simulink model "MdXXHolderChk"  (R2024b)
settings: Solver=FixedStepDiscrete  StartTime=0.0  StopTime=10.0  FixedStep=0.01  RelTol=1e-3
undefined symbols (not defined in the file or in its folder): KeSMSwAcsMd32SecRwLtStBkReclnUpwdDnwdPos1_Val, KeSMSwAcsMd53SecRwRtStBkReclnUpwdDnwdPos1_Val, SeatChldLkSt
libraries: simulink x41
(part 1 of 5)
settings Model: Creator=sn2xws  LastModifiedBy=sn55gm
settings Model: ModifiedHistory=|
  | 2024.7.9 V3.0.0 557模式流程V1.9
  | 2024.8.22 V3.0.1 修改Md8 Md9 退出逻辑
  | 2024.8.27 V3.0.2 Md1退出逻辑增加
  | 2024.8.28 V3.0.3 修正设置的bit位
  | 2024.10.25 V3.0.4 6s版 vipR不看三左儿童锁
  | 2024.10.29 V3.0.5 新增三排儿童锁逻辑
  | 2024.11.20 V3.0.6 md8，md9 只有7s版本需要看二排儿童锁
  | 2024.11.26 V3.0.7 Md28 只有7s版本需要看三排左儿童锁，Md27需要看三排童锁
  | 2024.12.11 V3.0.8 CR955881
  | 2024.12.23 V3.8.0 CR963463 二三排复位模式和大四座模式调用前提条件优化
  | 2025.3.5 V3.9.0 Bug 998190 7s 2L儿童锁Lock状态，2L靠背为0%，2R靠背大于31.7%，VCU调用mode 8，StPassCmprtMd_Md8_VCU_RclRspStat= error（应为successfully）
  | 2025.5.13 V3.12.0 Md11，md13，md32,md53童锁条件遗漏
  | 2025.5.14 V3.12.1 bug 1038602童锁时不应该动靠背
  | 2025.5.20 V3.12.2 bug 1038602童锁时不应该动靠背
  | 25.7.2 V3.13.0 新增Md61 Md62
settings SolverCC: AlgebraicLoopSolver=TrustRegion
settings DataIOCC: SaveFormat=StructureWithTime  ReturnWorkspaceOutputs=off
settings OptimizationCC: DefaultParameterBehavior=Inlined  EnhancedBackFolding=on  PassReuseOutputArgsAs=Individual arguments  ZeroExternalMemoryAtStartup=off  ZeroInternalMemoryAtStartup=off  OptimizeBlockOrder=speed  DifferentSizesBufferReuse=on  OptimizationCustomize=off  EfficientTunableParamExpr=on
settings DebuggingCC: ParameterTunabilityLossMsg=error  UnconnectedInputMsg=warning  UnconnectedOutputMsg=warning  UnconnectedLineMsg=warning  ArithmeticOperatorsInVariantConditions=warning
settings ModelReferenceCC: EnableRefExpFcnMdlSchedulingChecks=on
settings SFSimCC: MATLABDynamicMemAlloc=off  CustomCodeUndefinedFunction=UseInterfaceOnly
settings RTWCC: Description=AUTOSAR  SystemTargetFile=autosar.tlc  GenCodeOnly=on  TemplateMakefile=ert_default_tmf  GenerateReport=on  IncludeHyperlinkInReport=on  LaunchReport=on  DataTypeReplacement=CDataTypesFixedWidth  GenerateTraceInfo=on  GenerateTraceReport=on  GenerateTraceReportSl=on  GenerateTraceReportSf=on  GenerateTraceReportEml=on  GPUComputeCapability=3.5
settings CodeAppCC: ForceParamTrailComments=on  IgnoreCustomStorageClasses=off  OperatorAnnotations=on  SimulinkDataObjDesc=on  SFDataObjDesc=on  InsertBlockDesc=on
settings STFCustomTargetCC: TargetLangStandard=C99 (ISO)  MultiwordLength=256  ParMdlRefBuildCompliant=on  CompOptLevelCompliant=on  IncludeMdlTerminateFcn=off  CombineOutputUpdateFcns=on  SuppressErrorStatus=on  ERTCustomFileBanners=on  SupportNonFinite=off  SupportComplex=off  SupportContinuousTime=off  SupportNonInlinedSFcns=off  RemoveResetFunc=on  MATLABClassNameForMDSCustomization=Simulink.SoftwareTarget.ERTCustomization  AutosarCompliant=on  UseToolchainInfoCompliant=on  LookupTableObjectStructAxisOrder=2,1,3,4,...  LUTObjectStructOrderEvenSpacing=Size,Table,Breakpoints  SystemTargetFile=autosar.tlc
settings ERTTargetCC: TargetLangStandard=C99 (ISO)  ConcurrentExecutionCompliant=off  IncludeMdlTerminateFcn=off  SuppressErrorStatus=on  SupportNonFinite=off  SupportComplex=off  ModelStepFunctionPrototypeControlCompliant=off  CPPClassGenCompliant=off  AutosarCompliant=on  LookupTableObjectStructAxisOrder=2,1,3,4,...  LUTObjectStructOrderEvenSpacing=Size,Table,Breakpoints  ERTCustomFileTemplate=example_file_process.tlc  ERTFilePackagingFormat=Compact  BooleanTrueId=TRUE  BooleanFalseId=FALSE  DynamicArrayContainerType=coder::array

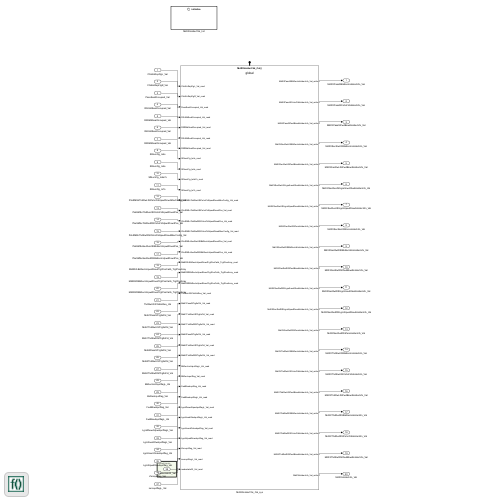
[thumbnail: Simulink's stored preview of the top-level diagram]
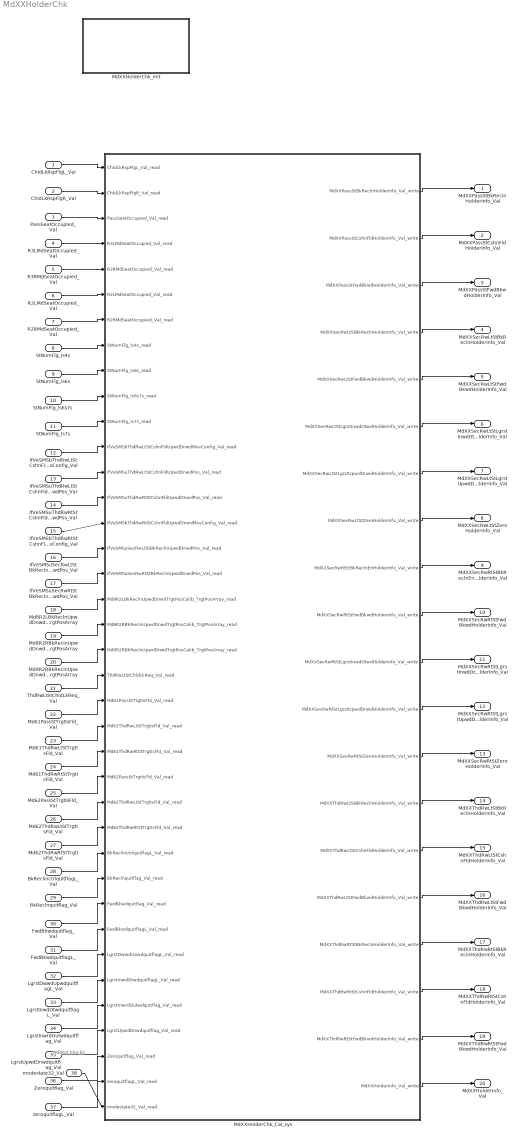
== system MdXXHolderChk ==
  note: Added blocks
  ChldLkRspFlgL_Val : Inport  OutDataTypeStr=boolean  PortDimensions=1
  ChldLkRspFlgR_Val : Inport  Port=2  OutDataTypeStr=boolean  PortDimensions=1
  PassSeatOccupied_Val : Inport  Port=3  OutDataTypeStr=boolean  PortDimensions=1
  R3LMdSeatOccupied_Val : Inport  Port=4  OutDataTypeStr=boolean  PortDimensions=1
  R3RMdSeatOccupied_Val : Inport  Port=5  OutDataTypeStr=boolean  PortDimensions=1
  R2LMdSeatOccupied_Val : Inport  Port=6  OutDataTypeStr=boolean  PortDimensions=1
  R2RMdSeatOccupied_Val : Inport  Port=7  OutDataTypeStr=boolean  PortDimensions=1
  StNumFlg_Is4s : Inport  Port=8  OutDataTypeStr=boolean  PortDimensions=1
  StNumFlg_Is6s : Inport  Port=9  OutDataTypeStr=boolean  PortDimensions=1
  StNumFlg_Is6s7s : Inport  Port=10  OutDataTypeStr=boolean  PortDimensions=1
  StNumFlg_Is7s : Inport  Port=11  OutDataTypeStr=boolean  PortDimensions=1
  IfVeSMSbThdRwLtStCshnFldUpwdDnwdMovConfig_Val : Inport  Port=12  OutDataTypeStr=boolean  PortDimensions=1
  IfVeSMSuThdRwLtStCshnFldUpwdDnwdPos_Val : Inport  Port=13  OutDataTypeStr=uint16  PortDimensions=1
  IfVeSMSuThdRwRtStCshnFldUpwdDnwdPos_Val : Inport  Port=14  OutDataTypeStr=uint16  PortDimensions=1
  IfVeSMSbThdRwRtStCshnFldUpwdDnwdMovConfig_Val : Inport  Port=15  OutDataTypeStr=boolean  PortDimensions=1
  IfVeSMSuSecRwLtStBkReclnUpwdDnwdPos_Val : Inport  Port=16  OutDataTypeStr=uint16  PortDimensions=1
  IfVeSMSuSecRwRtStBkReclnUpwdDnwdPos_Val : Inport  Port=17  OutDataTypeStr=uint16  PortDimensions=1
  Md8R2LBkReclnUpwdDnwdTrgtPosCalib_TrgtPosArray : Inport  Description=|  Port=18  OutDataTypeStr=uint16  PortDimensions=3
      | 0:Pos
      | 1:Max
      | 2:Min
  Md8R2RBkReclnUpwdDnwdTrgtPosCalib_TrgtPosArray : Inport  Description=|  Port=19  OutDataTypeStr=uint16  PortDimensions=3
      | 0:Pos
      | 1:Max
      | 2:Min
  Md9R2RBkReclnUpwdDnwdTrgtPosCalib_TrgtPosArray : Inport  Description=|  Port=20  OutDataTypeStr=uint16  PortDimensions=3
      | 0:Pos
      | 1:Max
      | 2:Min
  ThdRwLtStChldLkReq_Val : Inport  Port=21  OutDataTypeStr=Enum: SeatChldLkSt  PortDimensions=1
  Md61PassStTrgtIsFld_Val : Inport  Port=22  OutDataTypeStr=boolean  PortDimensions=1
  Md61ThdRwLtStTrgtIsFld_Val : Inport  Port=23  OutDataTypeStr=boolean  PortDimensions=1
  Md61ThdRwRtStTrgtIsFld_Val : Inport  Port=24  OutDataTypeStr=boolean  PortDimensions=1
  Md62PassStTrgtIsFld_Val : Inport  Port=25  OutDataTypeStr=boolean  PortDimensions=1
  Md62ThdRwLtStTrgtIsFld_Val : Inport  Port=26  OutDataTypeStr=boolean  PortDimensions=1
  Md62ThdRwRtStTrgtIsFld_Val : Inport  Port=27  OutDataTypeStr=boolean  PortDimensions=1
  BkReclinctrlquitflagL_Val : Inport  Port=28  OutDataTypeStr=boolean  PortDimensions=1
  BkReclnquitflag_Val : Inport  Port=29  OutDataTypeStr=boolean  PortDimensions=1
  FwdBkwdquitflag_Val : Inport  Port=30  OutDataTypeStr=boolean  PortDimensions=1
  FwdBkwdquitflagL_Val : Inport  Port=31  OutDataTypeStr=boolean  PortDimensions=1
  LgrstDwwdUpwdquitflagL_Val : Inport  Port=32  OutDataTypeStr=boolean  PortDimensions=1
  LgrstInwdOtwdquitflagL_Val : Inport  Port=33  OutDataTypeStr=boolean  PortDimensions=1
  LgrstInwrdOutwdquitflag_Val : Inport  Port=34  OutDataTypeStr=boolean  PortDimensions=1
  LgrstUpwdDnwdquitflag_Val : Inport  Port=35  OutDataTypeStr=boolean  PortDimensions=1
  Zeroquitflag_Val : Inport  Port=36  OutDataTypeStr=boolean  PortDimensions=1
  zeroquitflagL_Val : Inport  Port=37  OutDataTypeStr=boolean  PortDimensions=1
  modestate32_Val : Inport  Port=38  OutDataTypeStr=uint32  PortDimensions=1
  MdXXHolderChk_Cal_sys : Subsystem
  MdXXHolderChk_Init : Subsystem
  MdXXPassStBkReclnHolderInfo_Val : Outport  OutDataTypeStr=uint32  PortDimensions=1  VectorParamsAs1DForOutWhenUnconnected=off
  MdXXPassStCshnFldHolderInfo_Val : Outport  Port=2  OutDataTypeStr=uint32  PortDimensions=1  VectorParamsAs1DForOutWhenUnconnected=off
  MdXXPassStFwdBkwdHolderInfo_Val : Outport  Port=3  OutDataTypeStr=uint32  PortDimensions=1  VectorParamsAs1DForOutWhenUnconnected=off
  MdXXSecRwLtStBkReclnHolderInfo_Val : Outport  Port=4  OutDataTypeStr=uint32  PortDimensions=1  VectorParamsAs1DForOutWhenUnconnected=off
  MdXXSecRwLtStFwdBkwdHolderInfo_Val : Outport  Port=5  OutDataTypeStr=uint32  PortDimensions=1  VectorParamsAs1DForOutWhenUnconnected=off
  MdXXSecRwLtStLgrstInwdOtwdHolderInfo_Val : Outport  Port=6  OutDataTypeStr=uint32  PortDimensions=1  VectorParamsAs1DForOutWhenUnconnected=off
  MdXXSecRwLtStLgrstUpwdDnwdHolderInfo_Val : Outport  Port=7  OutDataTypeStr=uint32  PortDimensions=1  VectorParamsAs1DForOutWhenUnconnected=off
  MdXXSecRwLtStZeroHolderInfo_Val : Outport  Port=8  OutDataTypeStr=uint32  PortDimensions=1  VectorParamsAs1DForOutWhenUnconnected=off
  MdXXSecRwRtStBkReclnEnHolderInfo_Val : Outport  Port=9  OutDataTypeStr=uint32  PortDimensions=1  VectorParamsAs1DForOutWhenUnconnected=off
  MdXXSecRwRtStFwdBkwdHolderInfo_Val : Outport  Port=10  OutDataTypeStr=uint32  PortDimensions=1  VectorParamsAs1DForOutWhenUnconnected=off
  MdXXSecRwRtStLgrstInwdOtwdHolderInfo_Val : Outport  Port=11  OutDataTypeStr=uint32  PortDimensions=1  VectorParamsAs1DForOutWhenUnconnected=off
  MdXXSecRwRtStLgrstUpwdDnwdHolderInfo_Val : Outport  Port=12  OutDataTypeStr=uint32  PortDimensions=1  VectorParamsAs1DForOutWhenUnconnected=off
  MdXXSecRwRtStZeroHolderInfo_Val : Outport  Port=13  OutDataTypeStr=uint32  PortDimensions=1  VectorParamsAs1DForOutWhenUnconnected=off
  MdXXThdRwLtStBkReclnHolderInfo_Val : Outport  Port=14  OutDataTypeStr=uint32  PortDimensions=1  VectorParamsAs1DForOutWhenUnconnected=off
  MdXXThdRwLtStCshnFldHolderInfo_Val : Outport  Port=15  OutDataTypeStr=uint32  PortDimensions=1  VectorParamsAs1DForOutWhenUnconnected=off
  MdXXThdRwLtStFwdBkwdHolderInfo_Val : Outport  Port=16  OutDataTypeStr=uint32  PortDimensions=1  VectorParamsAs1DForOutWhenUnconnected=off
  MdXXThdRwRtStBkReclnHolderInfo_Val : Outport  Port=17  OutDataTypeStr=uint32  PortDimensions=1  VectorParamsAs1DForOutWhenUnconnected=off
  MdXXThdRwRtStCshnFldHolderInfo_Val : Outport  Port=18  OutDataTypeStr=uint32  PortDimensions=1  VectorParamsAs1DForOutWhenUnconnected=off
  MdXXThdRwRtStFwdBkwdHolderInfo_Val : Outport  Port=19  OutDataTypeStr=uint32  PortDimensions=1  VectorParamsAs1DForOutWhenUnconnected=off
  MdXXHolderInfo_Val : Outport  Port=20  OutDataTypeStr=uint32  PortDimensions=1  VectorParamsAs1DForOutWhenUnconnected=off
  wires:
  ChldLkRspFlgL_Val/1 -> MdXXHolderChk_Cal_sys/1(ChldLkRspFlgL_Val_read)
  ChldLkRspFlgR_Val/1 -> MdXXHolderChk_Cal_sys/2(ChldLkRspFlgR_Val_read)
  PassSeatOccupied_Val/1 -> MdXXHolderChk_Cal_sys/3(PassSeatOccupied_Val_read)
  R3LMdSeatOccupied_Val/1 -> MdXXHolderChk_Cal_sys/4(R3LMdSeatOccupied_Val_read)
  R3RMdSeatOccupied_Val/1 -> MdXXHolderChk_Cal_sys/5(R3RMdSeatOccupied_Val_read)
  MdXXHolderChk_Cal_sys/1(MdXXPassStBkReclnHolderInfo_Val_write) -> MdXXPassStBkReclnHolderInfo_Val/1
  MdXXHolderChk_Cal_sys/2(MdXXPassStCshnFldHolderInfo_Val_write) -> MdXXPassStCshnFldHolderInfo_Val/1
  MdXXHolderChk_Cal_sys/3(MdXXPassStFwdBkwdHolderInfo_Val_write) -> MdXXPassStFwdBkwdHolderInfo_Val/1
  MdXXHolderChk_Cal_sys/4(MdXXSecRwLtStBkReclnHolderInfo_Val_write) -> MdXXSecRwLtStBkReclnHolderInfo_Val/1
  MdXXHolderChk_Cal_sys/5(MdXXSecRwLtStFwdBkwdHolderInfo_Val_write) -> MdXXSecRwLtStFwdBkwdHolderInfo_Val/1
  MdXXHolderChk_Cal_sys/6(MdXXSecRwLtStLgrstInwdOtwdHolderInfo_Val_write) -> MdXXSecRwLtStLgrstInwdOtwdHolderInfo_Val/1
  MdXXHolderChk_Cal_sys/7(MdXXSecRwLtStLgrstUpwdDnwdHolderInfo_Val_write) -> MdXXSecRwLtStLgrstUpwdDnwdHolderInfo_Val/1
  MdXXHolderChk_Cal_sys/8(MdXXSecRwLtStZeroHolderInfo_Val_write) -> MdXXSecRwLtStZeroHolderInfo_Val/1
  MdXXHolderChk_Cal_sys/9(MdXXSecRwRtStBkReclnEnHolderInfo_Val_write) -> MdXXSecRwRtStBkReclnEnHolderInfo_Val/1
  MdXXHolderChk_Cal_sys/10(MdXXSecRwRtStFwdBkwdHolderInfo_Val_write) -> MdXXSecRwRtStFwdBkwdHolderInfo_Val/1
  MdXXHolderChk_Cal_sys/11(MdXXSecRwRtStLgrstInwdOtwdHolderInfo_Val_write) -> MdXXSecRwRtStLgrstInwdOtwdHolderInfo_Val/1
  MdXXHolderChk_Cal_sys/12(MdXXSecRwRtStLgrstUpwdDnwdHolderInfo_Val_write) -> MdXXSecRwRtStLgrstUpwdDnwdHolderInfo_Val/1
  MdXXHolderChk_Cal_sys/13(MdXXSecRwRtStZeroHolderInfo_Val_write) -> MdXXSecRwRtStZeroHolderInfo_Val/1
  MdXXHolderChk_Cal_sys/14(MdXXThdRwLtStBkReclnHolderInfo_Val_write) -> MdXXThdRwLtStBkReclnHolderInfo_Val/1
  MdXXHolderChk_Cal_sys/15(MdXXThdRwLtStCshnFldHolderInfo_Val_write) -> MdXXThdRwLtStCshnFldHolderInfo_Val/1
  MdXXHolderChk_Cal_sys/16(MdXXThdRwLtStFwdBkwdHolderInfo_Val_write) -> MdXXThdRwLtStFwdBkwdHolderInfo_Val/1
  MdXXHolderChk_Cal_sys/17(MdXXThdRwRtStBkReclnHolderInfo_Val_write) -> MdXXThdRwRtStBkReclnHolderInfo_Val/1
  MdXXHolderChk_Cal_sys/18(MdXXThdRwRtStCshnFldHolderInfo_Val_write) -> MdXXThdRwRtStCshnFldHolderInfo_Val/1
  MdXXHolderChk_Cal_sys/19(MdXXThdRwRtStFwdBkwdHolderInfo_Val_write) -> MdXXThdRwRtStFwdBkwdHolderInfo_Val/1
  R2LMdSeatOccupied_Val/1 -> MdXXHolderChk_Cal_sys/6(R2LMdSeatOccupied_Val_read)
  R2RMdSeatOccupied_Val/1 -> MdXXHolderChk_Cal_sys/7(R2RMdSeatOccupied_Val_read)
  StNumFlg_Is4s/1 -> MdXXHolderChk_Cal_sys/8(StNumFlg_Is4s_read)
  StNumFlg_Is6s/1 -> MdXXHolderChk_Cal_sys/9(StNumFlg_Is6s_read)
  StNumFlg_Is6s7s/1 -> MdXXHolderChk_Cal_sys/10(StNumFlg_Is6s7s_read)
  StNumFlg_Is7s/1 -> MdXXHolderChk_Cal_sys/11(StNumFlg_Is7s_read)
  IfVeSMSbThdRwLtStCshnFldUpwdDnwdMovConfig_Val/1 -> MdXXHolderChk_Cal_sys/12(IfVeSMSbThdRwLtStCshnFldUpwdDnwdMovConfig_Val_read)
  IfVeSMSuThdRwLtStCshnFldUpwdDnwdPos_Val/1 -> MdXXHolderChk_Cal_sys/13(IfVeSMSuThdRwLtStCshnFldUpwdDnwdPos_Val_read)
  IfVeSMSuThdRwRtStCshnFldUpwdDnwdPos_Val/1 -> MdXXHolderChk_Cal_sys/14(IfVeSMSuThdRwRtStCshnFldUpwdDnwdPos_Val_read)
  IfVeSMSbThdRwRtStCshnFldUpwdDnwdMovConfig_Val/1 -> MdXXHolderChk_Cal_sys/15(IfVeSMSbThdRwRtStCshnFldUpwdDnwdMovConfig_Val_read)
  IfVeSMSuSecRwLtStBkReclnUpwdDnwdPos_Val/1 -> MdXXHolderChk_Cal_sys/16(IfVeSMSuSecRwLtStBkReclnUpwdDnwdPos_Val_read)
  IfVeSMSuSecRwRtStBkReclnUpwdDnwdPos_Val/1 -> MdXXHolderChk_Cal_sys/17(IfVeSMSuSecRwRtStBkReclnUpwdDnwdPos_Val_read)
  Md8R2LBkReclnUpwdDnwdTrgtPosCalib_TrgtPosArray/1 -> MdXXHolderChk_Cal_sys/18(Md8R2LBkReclnUpwdDnwdTrgtPosCalib_TrgtPosArray_read)
  Md8R2RBkReclnUpwdDnwdTrgtPosCalib_TrgtPosArray/1 -> MdXXHolderChk_Cal_sys/19(Md8R2RBkReclnUpwdDnwdTrgtPosCalib_TrgtPosArray_read)
  Md9R2RBkReclnUpwdDnwdTrgtPosCalib_TrgtPosArray/1 -> MdXXHolderChk_Cal_sys/20(Md9R2RBkReclnUpwdDnwdTrgtPosCalib_TrgtPosArray_read)
  ThdRwLtStChldLkReq_Val/1 -> MdXXHolderChk_Cal_sys/21(ThdRwLtStChldLkReq_Val_read)
  MdXXHolderChk_Cal_sys/20(MdXXHolderInfo_Val_write) -> MdXXHolderInfo_Val/1
  Md61PassStTrgtIsFld_Val/1 -> MdXXHolderChk_Cal_sys/22(Md61PassStTrgtIsFld_Val_read)
  Md61ThdRwLtStTrgtIsFld_Val/1 -> MdXXHolderChk_Cal_sys/23(Md61ThdRwLtStTrgtIsFld_Val_read)
  Md61ThdRwRtStTrgtIsFld_Val/1 -> MdXXHolderChk_Cal_sys/24(Md61ThdRwRtStTrgtIsFld_Val_read)
  Md62PassStTrgtIsFld_Val/1 -> MdXXHolderChk_Cal_sys/25(Md62PassStTrgtIsFld_Val_read)
  Md62ThdRwLtStTrgtIsFld_Val/1 -> MdXXHolderChk_Cal_sys/26(Md62ThdRwLtStTrgtIsFld_Val_read)
  Md62ThdRwRtStTrgtIsFld_Val/1 -> MdXXHolderChk_Cal_sys/27(Md62ThdRwRtStTrgtIsFld_Val_read)
  BkReclinctrlquitflagL_Val/1 -> MdXXHolderChk_Cal_sys/28(BkReclinctrlquitflagL_Val_read)
  BkReclnquitflag_Val/1 -> MdXXHolderChk_Cal_sys/29(BkReclnquitflag_Val_read)
  FwdBkwdquitflag_Val/1 -> MdXXHolderChk_Cal_sys/30(FwdBkwdquitflag_Val_read)
  FwdBkwdquitflagL_Val/1 -> MdXXHolderChk_Cal_sys/31(FwdBkwdquitflagL_Val_read)
  LgrstDwwdUpwdquitflagL_Val/1 -> MdXXHolderChk_Cal_sys/32(LgrstDwwdUpwdquitflagL_Val_read)
  LgrstInwdOtwdquitflagL_Val/1 -> MdXXHolderChk_Cal_sys/33(LgrstInwdOtwdquitflagL_Val_read)
  LgrstInwrdOutwdquitflag_Val/1 -> MdXXHolderChk_Cal_sys/34(LgrstInwrdOutwdquitflag_Val_read)
  LgrstUpwdDnwdquitflag_Val/1 -> MdXXHolderChk_Cal_sys/35(LgrstUpwdDnwdquitflag_Val_read)
  Zeroquitflag_Val/1 -> MdXXHolderChk_Cal_sys/36(Zeroquitflag_Val_read)
  zeroquitflagL_Val/1 -> MdXXHolderChk_Cal_sys/37(zeroquitflagL_Val_read)
  modestate32_Val/1 -> MdXXHolderChk_Cal_sys/38(modestate32_Val_read)

== system MdXXHolderChk/MdXXHolderChk_Cal_sys ==
  note: Added blocks
  note: Added blocks
  note: Added blocks
  ChldLkRspFlgL_Val_read : Inport
  ChldLkRspFlgR_Val_read : Inport  Port=2
  PassSeatOccupied_Val_read : Inport  Port=3
  R3LMdSeatOccupied_Val_read : Inport  Port=4
  R3RMdSeatOccupied_Val_read : Inport  Port=5
  R2LMdSeatOccupied_Val_read : Inport  Port=6
  R2RMdSeatOccupied_Val_read : Inport  Port=7
  StNumFlg_Is4s_read : Inport  Port=8
  StNumFlg_Is6s_read : Inport  Port=9
  StNumFlg_Is6s7s_read : Inport  Port=10
  StNumFlg_Is7s_read : Inport  Port=11
  IfVeSMSbThdRwLtStCshnFldUpwdDnwdMovConfig_Val_read : Inport  Port=12
  IfVeSMSuThdRwLtStCshnFldUpwdDnwdPos_Val_read : Inport  Port=13
  IfVeSMSuThdRwRtStCshnFldUpwdDnwdPos_Val_read : Inport  Port=14
  IfVeSMSbThdRwRtStCshnFldUpwdDnwdMovConfig_Val_read : Inport  Port=15
  IfVeSMSuSecRwLtStBkReclnUpwdDnwdPos_Val_read : Inport  Port=16
  IfVeSMSuSecRwRtStBkReclnUpwdDnwdPos_Val_read : Inport  Port=17
  Md8R2LBkReclnUpwdDnwdTrgtPosCalib_TrgtPosArray_read : Inport  Port=18
  Md8R2RBkReclnUpwdDnwdTrgtPosCalib_TrgtPosArray_read : Inport  Port=19
  Md9R2RBkReclnUpwdDnwdTrgtPosCalib_TrgtPosArray_read : Inport  Port=20
  ThdRwLtStChldLkReq_Val_read : Inport  Port=21
  Md61PassStTrgtIsFld_Val_read : Inport  Port=22
  Md61ThdRwLtStTrgtIsFld_Val_read : Inport  Port=23
  Md61ThdRwRtStTrgtIsFld_Val_read : Inport  Port=24
  Md62PassStTrgtIsFld_Val_read : Inport  Port=25
  Md62ThdRwLtStTrgtIsFld_Val_read : Inport  Port=26
  Md62ThdRwRtStTrgtIsFld_Val_read : Inport  Port=27
  BkReclinctrlquitflagL_Val_read : Inport  Port=28
  BkReclnquitflag_Val_read : Inport  Port=29
  FwdBkwdquitflag_Val_read : Inport  Port=30
  FwdBkwdquitflagL_Val_read : Inport  Port=31
  LgrstDwwdUpwdquitflagL_Val_read : Inport  Port=32
  LgrstInwdOtwdquitflagL_Val_read : Inport  Port=33
  LgrstInwrdOutwdquitflag_Val_read : Inport  Port=34
  LgrstUpwdDnwdquitflag_Val_read : Inport  Port=35
  Zeroquitflag_Val_read : Inport  Port=36
  zeroquitflagL_Val_read : Inport  Port=37
  modestate32_Val_read : Inport  Port=38
  function : TriggerPort  TriggerType=function-call  IsSimulinkFunction=on  FunctionName=MdXXHolderChk_Cal  VariantControl=(inherit)
  PA_KeSMSwAcsMd32SecRwLtStBkReclnUpwdDnwdPos1_Val : Constant  Value=KeSMSwAcsMd32SecRwLtStBkReclnUpwdDnwdPos1_Val
  PA_KeSMSwAcsMd53SecRwRtStBkReclnUpwdDnwdPos1_Val : Constant  Value=KeSMSwAcsMd53SecRwRtStBkReclnUpwdDnwdPos1_Val
  Subsystem : Subsystem
  Terminator_1 : Terminator
  Terminator_2 : Terminator
  Terminator_3 : Terminator
  MdXXPassStBkReclnHolderInfo_Val_write : Outport  VectorParamsAs1DForOutWhenUnconnected=off
      settings: EnsureOutportIsVirtual=on
  MdXXPassStCshnFldHolderInfo_Val_write : Outport  Port=2  VectorParamsAs1DForOutWhenUnconnected=off
      settings: EnsureOutportIsVirtual=on
  MdXXPassStFwdBkwdHolderInfo_Val_write : Outport  Port=3  VectorParamsAs1DForOutWhenUnconnected=off
      settings: EnsureOutportIsVirtual=on
  MdXXSecRwLtStBkReclnHolderInfo_Val_write : Outport  Port=4  VectorParamsAs1DForOutWhenUnconnected=off
      settings: EnsureOutportIsVirtual=on
  MdXXSecRwLtStFwdBkwdHolderInfo_Val_write : Outport  Port=5  VectorParamsAs1DForOutWhenUnconnected=off
      settings: EnsureOutportIsVirtual=on
  MdXXSecRwLtStLgrstInwdOtwdHolderInfo_Val_write : Outport  Port=6  VectorParamsAs1DForOutWhenUnconnected=off
      settings: EnsureOutportIsVirtual=on
  MdXXSecRwLtStLgrstUpwdDnwdHolderInfo_Val_write : Outport  Port=7  VectorParamsAs1DForOutWhenUnconnected=off
      settings: EnsureOutportIsVirtual=on
  MdXXSecRwLtStZeroHolderInfo_Val_write : Outport  Port=8  VectorParamsAs1DForOutWhenUnconnected=off
      settings: EnsureOutportIsVirtual=on
  MdXXSecRwRtStBkReclnEnHolderInfo_Val_write : Outport  Port=9  VectorParamsAs1DForOutWhenUnconnected=off
      settings: EnsureOutportIsVirtual=on
  MdXXSecRwRtStFwdBkwdHolderInfo_Val_write : Outport  Port=10  VectorParamsAs1DForOutWhenUnconnected=off
      settings: EnsureOutportIsVirtual=on
  MdXXSecRwRtStLgrstInwdOtwdHolderInfo_Val_write : Outport  Port=11  VectorParamsAs1DForOutWhenUnconnected=off
      settings: EnsureOutportIsVirtual=on
  MdXXSecRwRtStLgrstUpwdDnwdHolderInfo_Val_write : Outport  Port=12  VectorParamsAs1DForOutWhenUnconnected=off
      settings: EnsureOutportIsVirtual=on
  MdXXSecRwRtStZeroHolderInfo_Val_write : Outport  Port=13  VectorParamsAs1DForOutWhenUnconnected=off
      settings: EnsureOutportIsVirtual=on
  MdXXThdRwLtStBkReclnHolderInfo_Val_write : Outport  Port=14  VectorParamsAs1DForOutWhenUnconnected=off
      settings: EnsureOutportIsVirtual=on
  MdXXThdRwLtStCshnFldHolderInfo_Val_write : Outport  Port=15  VectorParamsAs1DForOutWhenUnconnected=off
      settings: EnsureOutportIsVirtual=on
  MdXXThdRwLtStFwdBkwdHolderInfo_Val_write : Outport  Port=16  VectorParamsAs1DForOutWhenUnconnected=off
      settings: EnsureOutportIsVirtual=on
  MdXXThdRwRtStBkReclnHolderInfo_Val_write : Outport  Port=17  VectorParamsAs1DForOutWhenUnconnected=off
      settings: EnsureOutportIsVirtual=on
  MdXXThdRwRtStCshnFldHolderInfo_Val_write : Outport  Port=18  VectorParamsAs1DForOutWhenUnconnected=off
      settings: EnsureOutportIsVirtual=on
  MdXXThdRwRtStFwdBkwdHolderInfo_Val_write : Outport  Port=19  VectorParamsAs1DForOutWhenUnconnected=off
      settings: EnsureOutportIsVirtual=on
  MdXXHolderInfo_Val_write : Outport  Port=20  VectorParamsAs1DForOutWhenUnconnected=off
      settings: EnsureOutportIsVirtual=on
  wires:
  ChldLkRspFlgL_Val_read/1 -> Subsystem/1(ChldLkRspFlgL_Val_read)
  ChldLkRspFlgR_Val_read/1 -> Subsystem/2(ChldLkRspFlgR_Val_read)
  PassSeatOccupied_Val_read/1 -> Subsystem/3(PassSeatOccupied_Val_read)
  R3LMdSeatOccupied_Val_read/1 -> Subsystem/4(R3LMdSeatOccupied_Val_read)
  R3RMdSeatOccupied_Val_read/1 -> Subsystem/5(R3RMdSeatOccupied_Val_read)
  Subsystem/1(MdXXPassStBkReclnHolderInfo_Val_write) -> MdXXPassStBkReclnHolderInfo_Val_write/1
  Subsystem/2(MdXXPassStCshnFldHolderInfo_Val_write) -> MdXXPassStCshnFldHolderInfo_Val_write/1
  Subsystem/3(MdXXPassStFwdBkwdHolderInfo_Val_write) -> MdXXPassStFwdBkwdHolderInfo_Val_write/1
  Subsystem/4(MdXXSecRwLtStBkReclnHolderInfo_Val_write) -> MdXXSecRwLtStBkReclnHolderInfo_Val_write/1
  Subsystem/5(MdXXSecRwLtStFwdBkwdHolderInfo_Val_write) -> MdXXSecRwLtStFwdBkwdHolderInfo_Val_write/1
  Subsystem/6(MdXXSecRwLtStLgrstInwdOtwdHolderInfo_Val_write) -> MdXXSecRwLtStLgrstInwdOtwdHolderInfo_Val_write/1
  Subsystem/7(MdXXSecRwLtStLgrstUpwdDnwdHolderInfo_Val_write) -> MdXXSecRwLtStLgrstUpwdDnwdHolderInfo_Val_write/1
  Subsystem/8(MdXXSecRwLtStZeroHolderInfo_Val_write) -> MdXXSecRwLtStZeroHolderInfo_Val_write/1
  Subsystem/9(MdXXSecRwRtStBkReclnEnHolderInfo_Val_write) -> MdXXSecRwRtStBkReclnEnHolderInfo_Val_write/1
  Subsystem/10(MdXXSecRwRtStFwdBkwdHolderInfo_Val_write) -> MdXXSecRwRtStFwdBkwdHolderInfo_Val_write/1
  Subsystem/11(MdXXSecRwRtStLgrstInwdOtwdHolderInfo_Val_write) -> MdXXSecRwRtStLgrstInwdOtwdHolderInfo_Val_write/1
  Subsystem/12(MdXXSecRwRtStLgrstUpwdDnwdHolderInfo_Val_write) -> MdXXSecRwRtStLgrstUpwdDnwdHolderInfo_Val_write/1
  Subsystem/13(MdXXSecRwRtStZeroHolderInfo_Val_write) -> MdXXSecRwRtStZeroHolderInfo_Val_write/1
  Subsystem/14(MdXXThdRwLtStBkReclnHolderInfo_Val_write) -> MdXXThdRwLtStBkReclnHolderInfo_Val_write/1
  Subsystem/15(MdXXThdRwLtStCshnFldHolderInfo_Val_write) -> MdXXThdRwLtStCshnFldHolderInfo_Val_write/1
  Subsystem/16(MdXXThdRwLtStFwdBkwdHolderInfo_Val_write) -> MdXXThdRwLtStFwdBkwdHolderInfo_Val_write/1
  Subsystem/17(MdXXThdRwRtStBkReclnHolderInfo_Val_write) -> MdXXThdRwRtStBkReclnHolderInfo_Val_write/1
  Subsystem/18(MdXXThdRwRtStCshnFldHolderInfo_Val_write) -> MdXXThdRwRtStCshnFldHolderInfo_Val_write/1
  Subsystem/19(MdXXThdRwRtStFwdBkwdHolderInfo_Val_write) -> MdXXThdRwRtStFwdBkwdHolderInfo_Val_write/1
  R2LMdSeatOccupied_Val_read/1 -> Subsystem/6(R2LMdSeatOccupied_Val_read)
  R2RMdSeatOccupied_Val_read/1 -> Subsystem/7(R2RMdSeatOccupied_Val_read)
  StNumFlg_Is4s_read/1 -> Terminator_1/1
  StNumFlg_Is6s_read/1 -> Terminator_2/1
  StNumFlg_Is6s7s_read/1 -> Terminator_3/1
  StNumFlg_Is7s_read/1 -> Subsystem/8(StNumFlg_Is7s_read)
  IfVeSMSbThdRwLtStCshnFldUpwdDnwdMovConfig_Val_read/1 -> Subsystem/9(IfVeSMSbThdRwLtStCshnFldUpwdDnwdMovConfig_Val_read)
  IfVeSMSuThdRwLtStCshnFldUpwdDnwdPos_Val_read/1 -> Subsystem/10(IfVeSMSuThdRwLtStCshnFldUpwdDnwdPos_Val_read)
  IfVeSMSuThdRwRtStCshnFldUpwdDnwdPos_Val_read/1 -> Subsystem/11(IfVeSMSuThdRwRtStCshnFldUpwdDnwdPos_Val_read)
  IfVeSMSbThdRwRtStCshnFldUpwdDnwdMovConfig_Val_read/1 -> Subsystem/12(IfVeSMSbThdRwRtStCshnFldUpwdDnwdMovConfig_Val_read)
  IfVeSMSuSecRwLtStBkReclnUpwdDnwdPos_Val_read/1 -> Subsystem/13(IfVeSMSuSecRwLtStBkReclnUpwdDnwdPos_Val_read)
  IfVeSMSuSecRwRtStBkReclnUpwdDnwdPos_Val_read/1 -> Subsystem/14(IfVeSMSuSecRwRtStBkReclnUpwdDnwdPos_Val_read)
  Md8R2LBkReclnUpwdDnwdTrgtPosCalib_TrgtPosArray_read/1 -> Subsystem/15(Md8R2LBkReclnUpwdDnwdTrgtPosCalib_TrgtPosArray_read)
  Md8R2RBkReclnUpwdDnwdTrgtPosCalib_TrgtPosArray_read/1 -> Subsystem/16(Md8R2RBkReclnUpwdDnwdTrgtPosCalib_TrgtPosArray_read)
  Md9R2RBkReclnUpwdDnwdTrgtPosCalib_TrgtPosArray_read/1 -> Subsystem/17(Md9R2RBkReclnUpwdDnwdTrgtPosCalib_TrgtPosArray_read)
  ThdRwLtStChldLkReq_Val_read/1 -> Subsystem/18(ThdRwLtStChldLkReq_Val_read)
  Subsystem/20(MdXXHolderInfo_Val_write) -> MdXXHolderInfo_Val_write/1
  PA_KeSMSwAcsMd32SecRwLtStBkReclnUpwdDnwdPos1_Val/1 -> Subsystem/19(KeSMSwAcsMd32SecRwLtStBkReclnUpwdDnwdPos1)
  PA_KeSMSwAcsMd53SecRwRtStBkReclnUpwdDnwdPos1_Val/1 -> Subsystem/20(KeSMSwAcsMd53SecRwRtStBkReclnUpwdDnwdPos1)
  Md61PassStTrgtIsFld_Val_read/1 -> Subsystem/21(Md61PassStTrgtIsFld_Val_read)
  Md61ThdRwLtStTrgtIsFld_Val_read/1 -> Subsystem/22(Md61ThdRwLtStTrgtIsFld_Val_read)
  Md61ThdRwRtStTrgtIsFld_Val_read/1 -> Subsystem/23(Md61ThdRwRtStTrgtIsFld_Val_read)
  Md62PassStTrgtIsFld_Val_read/1 -> Subsystem/24(Md62PassStTrgtIsFld_Val_read)
  Md62ThdRwLtStTrgtIsFld_Val_read/1 -> Subsystem/25(Md62ThdRwLtStTrgtIsFld_Val_read)
  Md62ThdRwRtStTrgtIsFld_Val_read/1 -> Subsystem/26(Md62ThdRwRtStTrgtIsFld_Val_read)
  BkReclinctrlquitflagL_Val_read/1 -> Subsystem/27(BkReclinctrlquitflagL_Val_read)
  BkReclnquitflag_Val_read/1 -> Subsystem/28(BkReclnquitflag_Val_read)
  FwdBkwdquitflag_Val_read/1 -> Subsystem/29(FwdBkwdquitflag_Val_read)
  FwdBkwdquitflagL_Val_read/1 -> Subsystem/30(FwdBkwdquitflagL_Val_read)
  LgrstDwwdUpwdquitflagL_Val_read/1 -> Subsystem/31(LgrstDwwdUpwdquitflagL_Val_read)
  LgrstInwdOtwdquitflagL_Val_read/1 -> Subsystem/32(LgrstInwdOtwdquitflagL_Val_read)
  LgrstInwrdOutwdquitflag_Val_read/1 -> Subsystem/33(LgrstInwrdOutwdquitflag_Val_read)
  LgrstUpwdDnwdquitflag_Val_read/1 -> Subsystem/34(LgrstUpwdDnwdquitflag_Val_read)
  Zeroquitflag_Val_read/1 -> Subsystem/35(Zeroquitflag_Val_read)
  zeroquitflagL_Val_read/1 -> Subsystem/36(zeroquitflagL_Val_read)
  modestate32_Val_read/1 -> Subsystem/37(modestate32_Val_read)

== system MdXXHolderChk/MdXXHolderChk_Init ==
  note: Added blocks
  note: Added blocks
  Event Listener : EventListener  EventName=reset
  PA_KeSMSwAcsMd32SecRwLtStBkReclnUpwdDnwdPos1_Val : Constant  Value=KeSMSwAcsMd32SecRwLtStBkReclnUpwdDnwdPos1_Val
  PA_KeSMSwAcsMd53SecRwRtStBkReclnUpwdDnwdPos1_Val : Constant  Value=KeSMSwAcsMd53SecRwRtStBkReclnUpwdDnwdPos1_Val
  Terminator_1 : Terminator
  Terminator_2 : Terminator
  wires:
  PA_KeSMSwAcsMd32SecRwLtStBkReclnUpwdDnwdPos1_Val/1 -> Terminator_1/1
  PA_KeSMSwAcsMd53SecRwRtStBkReclnUpwdDnwdPos1_Val/1 -> Terminator_2/1
